simulink model "controle_motor_2"  (R2025a)
settings: Solver=ode23tb  StartTime=0.0  StopTime=60  MaxStep=1e-3  MinStep=1e-6  RelTol=1e-4
undefined symbols (not defined in the file): B, C, J, kic, kis, kpc, kps, L_a, R_a
libraries: simulink x2, spsPWMGeneratorDCDCLib x2, spspowerguiLib x1
settings Model: Creator=Keslley  LastModifiedBy=Keslley

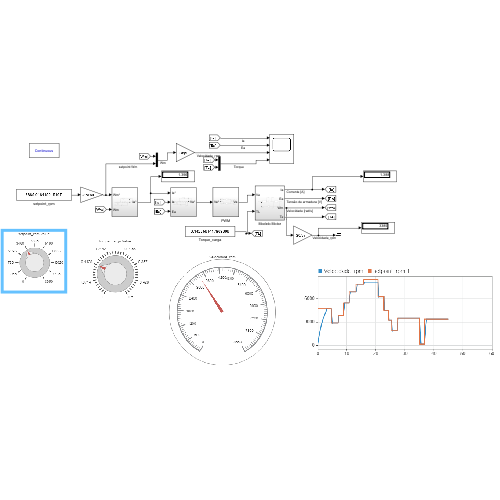
[thumbnail: Simulink's stored preview of the top-level diagram]
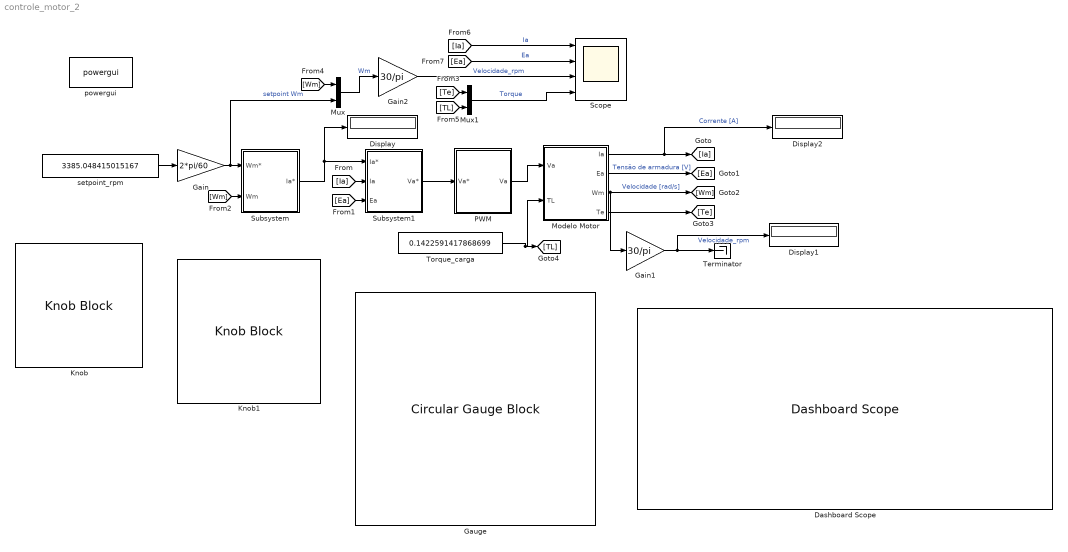
== system controle_motor_2 ==
  Dashboard Scope : DashboardScope  Ymin=0  Ymax=8650  FontColor=[0.0, 0.0, 0.0]
  Display : Display
  Display1 : Display
  Display2 : Display
  Gain : Gain  Gain=2*pi/60
  Gain1 : Gain  Gain=30/pi
  Gain2 : Gain  Gain=30/pi
  Gauge : CircularGaugeBlock  ScaleMax=8650  FontColor=[0.0, 0.0, 0.0]
  Knob : KnobBlock  ScaleMax=8650
  Knob1 : KnobBlock  ScaleMax=0.5
  Modelo Motor : Subsystem
  Mux : Mux  Inputs=2
  Mux1 : Mux  Inputs=2
  PWM : Subsystem
  Scope : Scope  NumInputPorts=4
      settings: ActiveDisplayYMinimum=-1797.4029531738308  ActiveDisplayYMaximum=9343.7536030720385
  Subsystem : Subsystem
  Subsystem1 : Subsystem
  Terminator : Terminator
  Torque_carga : Constant  Value=0.1422591417868699
  powergui : spspowerguiLib/powergui  Priority=1  SimulationMode=Continuous  SampleTime=50e-6  frequency=60  Iterations=50  frequencyindice=60  Pbase=100e6  ErrMax=1e-4  UnitsV=kV  UnitsW=MW  buscounter=0  FunctionMessages=off  echomessages=off  EnableUseOfTLC=off  CurrentSourceSwitches=off  DisableSnubberDevices=off  DisableRonSwitches=off  DisableVfSwitches=off  DisplayEquations=off  AutomaticDiscreteSolvers=off  SolverType=Tustin/Backward Euler (TBE)  Interpol=off  ExternalGateDelay=off  methode=off  Ts=100  x0status=blocks  SPID=on  SwTol=0  HookPort=off  NonlinearTolerance=1e-4  nMaxIteration=100  ContinueOnMaxIteration=off  RestoreLinks=warning  ResistiveCurrentMeasurement=off  Frange=[0:2:500]  Ylog=off  Xlog=on  ShowGrid=off  save=off  variable=ZData  structure=0  ZoomFFT=off  StartTime=0.0  cycles=1  DisplayStyle=1  fundamental=60  FreqAxis=off  MaxFrequency=1000  frequencyindicesteady=1  RmsSteady=1  display=off
  setpoint_rpm : Constant  Value=3385.048415015167
  wires:
  setpoint_rpm/1 -> Gain/1
  Gain/1 -> Mux/2, Subsystem/1(Wm*)  "setpoint Wm"
  Subsystem/1(Ia*) -> Display/1, Subsystem1/1(Ia*)
  [Ia] -> Subsystem1/2(Ia)
  [Ea] -> Subsystem1/3(Ea)
  Subsystem1/1(Va*) -> PWM/1(Va*)
  PWM/1(Va) -> Modelo Motor/1(Va)
  Torque_carga/1 -> Modelo Motor/2(TL), [TL]
  Modelo Motor/2(Ea) -> [Ea]  "Tensão de armadura [V]"
  Modelo Motor/1(Ia) -> Display2/1, [Ia]  "Corrente [A]"
  Modelo Motor/3(Wm) -> Gain1/1, [Wm]  "Velocidade [rad/s]"
  Modelo Motor/4(Te) -> [Te]
  Gain1/1 -> Display1/1, Terminator/1  "Velocidade_rpm"
  [Wm] -> Subsystem/2(Wm)
  [Wm] -> Mux/1
  Mux1/1 -> Scope/4  "Torque"
  [Te] -> Mux1/1
  [TL] -> Mux1/2
  [Ia] -> Scope/1  "Ia"
  [Ea] -> Scope/2  "Ea"
  Mux/1 -> Gain2/1  "Wm"
  Gain2/1 -> Scope/3  "Velocidade_rpm"

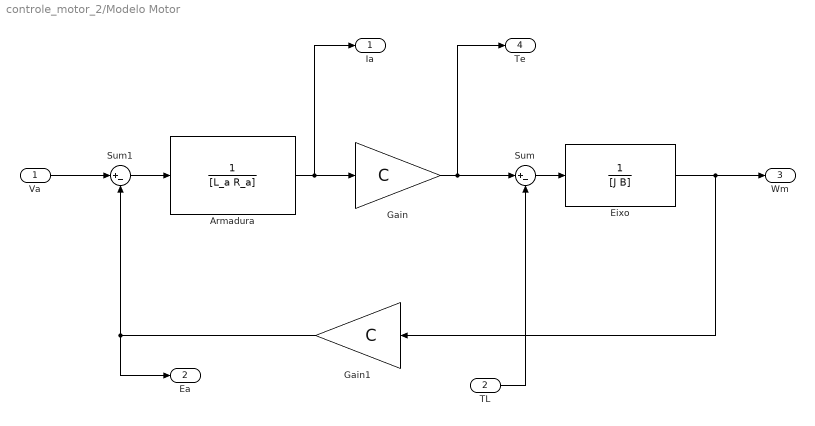
== system controle_motor_2/Modelo Motor ==
  Va : Inport
  TL : Inport  Port=2
  Armadura : TransferFcn  Denominator=[L_a R_a]
  Eixo : TransferFcn  Denominator=[J B]
  Gain : Gain  Gain=C
  Gain1 : Gain  Gain=C
  Sum : Sum  Inputs=|+-
  Sum1 : Sum  Inputs=|+-
  Ia : Outport  VectorParamsAs1DForOutWhenUnconnected=off
  Ea : Outport  Port=2  VectorParamsAs1DForOutWhenUnconnected=off
  Wm : Outport  Port=3  VectorParamsAs1DForOutWhenUnconnected=off
  Te : Outport  Port=4  VectorParamsAs1DForOutWhenUnconnected=off
  wires:
  Armadura/1 -> Ia/1, Gain/1
  Gain/1 -> Sum/1, Te/1
  Sum/1 -> Eixo/1
  Sum1/1 -> Armadura/1
  Va/1 -> Sum1/1
  Gain1/1 -> Ea/1, Sum1/2
  Eixo/1 -> Gain1/1, Wm/1
  TL/1 -> Sum/2

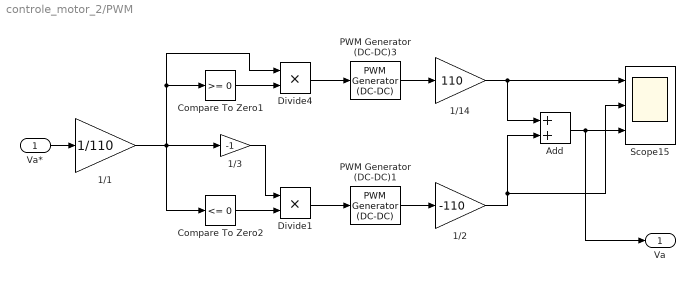
== system controle_motor_2/PWM ==
  Va* : Inport
  1/1 : Gain  Gain=1/110  SaturateOnIntegerOverflow=on  OutDataTypeStr=Inherit: Same as input  ParamDataTypeStr=Inherit: Same as input
  1/14 : Gain  Gain=110  SaturateOnIntegerOverflow=on  OutDataTypeStr=Inherit: Same as input  ParamDataTypeStr=Inherit: Same as input
  1/2 : Gain  Gain=-110  SaturateOnIntegerOverflow=on  OutDataTypeStr=Inherit: Same as input  ParamDataTypeStr=Inherit: Same as input
  1/3 : Gain  Gain=-1  SaturateOnIntegerOverflow=on  OutDataTypeStr=Inherit: Same as input  ParamDataTypeStr=Inherit: Same as input
  Add : Sum
  Compare To Zero1 : simulink/Logic and Bit Operations/Compare To Zero  relop=>=  OutDataTypeStr=boolean
  Compare To Zero2 : simulink/Logic and Bit Operations/Compare To Zero  relop=<=  OutDataTypeStr=boolean
  Divide1 : Product  Inputs=**
  Divide4 : Product  Inputs=**
  PWM Generator (DC-DC)1 : spsPWMGeneratorDCDCLib/PWM Generator (DC-DC)  Fsw=5000  Ts=0
  PWM Generator (DC-DC)3 : spsPWMGeneratorDCDCLib/PWM Generator (DC-DC)  Fsw=5000  Ts=0
  Scope15 : Scope  NumInputPorts=3
      settings: ActiveDisplayYMinimum=-1  ActiveDisplayYMaximum=1  DataLoggingVariableName=ScopeData7
  Va : Outport  InitialOutput=0
  wires:
  1/1/1 -> Compare To Zero2/1, 1/3/1, Compare To Zero1/1, Divide4/1
  Divide4/1 -> PWM Generator (DC-DC)3/1
  1/14/1 -> Add/1, Scope15/1
  PWM Generator (DC-DC)3/1 -> 1/14/1
  Compare To Zero1/1 -> Divide4/2
  Va*/1 -> 1/1/1
  PWM Generator (DC-DC)1/1 -> 1/2/1
  Compare To Zero2/1 -> Divide1/2
  Divide1/1 -> PWM Generator (DC-DC)1/1
  1/3/1 -> Divide1/1
  1/2/1 -> Scope15/2, Add/2
  Add/1 -> Scope15/3, Va/1

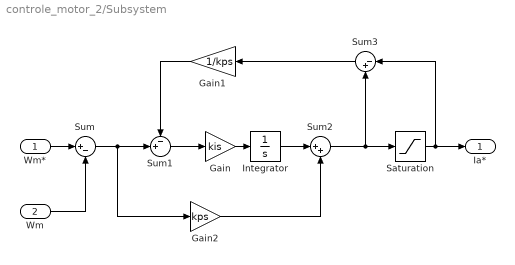
== system controle_motor_2/Subsystem ==
  Wm* : Inport
  Wm : Inport  Port=2
  Gain : Gain  Gain=kis
  Gain1 : Gain  Gain=1/kps
  Gain2 : Gain  Gain=kps
  Integrator : Integrator
  Saturation : Saturate  UpperLimit=2  LowerLimit=0
  Sum : Sum  Inputs=|+-
  Sum1 : Sum  Inputs=-+|
  Sum2 : Sum  Inputs=|++
  Sum3 : Sum  Inputs=|-+
  Ia* : Outport
  wires:
  Wm/1 -> Sum/2
  Wm*/1 -> Sum/1
  Sum/1 -> Gain2/1, Sum1/2
  Sum1/1 -> Gain/1
  Gain1/1 -> Sum1/1
  Gain/1 -> Integrator/1
  Integrator/1 -> Sum2/1
  Gain2/1 -> Sum2/2
  Sum2/1 -> Saturation/1, Sum3/2
  Saturation/1 -> Sum3/1, Ia*/1
  Sum3/1 -> Gain1/1

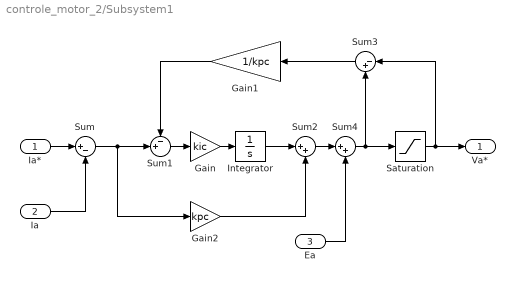
== system controle_motor_2/Subsystem1 ==
  Ia* : Inport
  Ia : Inport  Port=2
  Ea : Inport  Port=3
  Gain : Gain  Gain=kic
  Gain1 : Gain  Gain=1/kpc
  Gain2 : Gain  Gain=kpc
  Integrator : Integrator
  Saturation : Saturate  UpperLimit=110  LowerLimit=0
  Sum : Sum  Inputs=|+-
  Sum1 : Sum  Inputs=-+|
  Sum2 : Sum  Inputs=|++
  Sum3 : Sum  Inputs=|-+
  Sum4 : Sum  Inputs=|++
  Va* : Outport
  wires:
  Ia/1 -> Sum/2
  Ia*/1 -> Sum/1
  Sum/1 -> Gain2/1, Sum1/2
  Sum1/1 -> Gain/1
  Gain1/1 -> Sum1/1
  Gain/1 -> Integrator/1
  Integrator/1 -> Sum2/1
  Gain2/1 -> Sum2/2
  Saturation/1 -> Sum3/1, Va*/1
  Sum3/1 -> Gain1/1
  Sum2/1 -> Sum4/1
  Sum4/1 -> Sum3/2, Saturation/1
  Ea/1 -> Sum4/2
